simulink model "manipRotationTrajectory"  (R2019a)
settings: Solver=FixedStepAuto  StartTime=0.0  StopTime=inf  RelTol=1e-3
PreLoadFcn:
  | createWaypointData;
undefined symbols (not defined in the file): diff, gen3, maxWaypoints, ts, waypointTimes
libraries: trajExampleUtils x9, robotcorelib x4, robotmaniplib x1
settings Model: Creator=scastro  LastModifiedBy=scastro
settings DataIOCC: ReturnWorkspaceOutputs=off
settings OptimizationCC: DefaultParameterBehavior=Inlined  EnhancedBackFolding=on  PassReuseOutputArgsAs=Individual arguments  OptimizeBlockOrder=speed  DifferentSizesBufferReuse=on  OptimizationCustomize=off
settings DebuggingCC: ParameterTunabilityLossMsg=error  ArithmeticOperatorsInVariantConditions=warning
settings SFSimCC: MATLABDynamicMemAlloc=off
settings RTWCC: SystemTargetFile=ert.tlc  TemplateMakefile=ert_default_tmf  GenerateReport=on  IncludeHyperlinkInReport=on  LaunchReport=on  GenerateTraceInfo=on  GenerateTraceReport=on  GenerateTraceReportSl=on  GenerateTraceReportSf=on  GenerateTraceReportEml=on
settings CodeAppCC: ForceParamTrailComments=on  IgnoreCustomStorageClasses=off  OperatorAnnotations=on  SimulinkDataObjDesc=on  SFDataObjDesc=on  InsertBlockDesc=on
settings ERTTargetCC: TargetLangStandard=C99 (ISO)  GenerateSampleERTMain=on  SupportVariableSizeSignals=on  InlinedParameterPlacement=NonHierarchical  ERTCustomFileTemplate=example_file_process.tlc

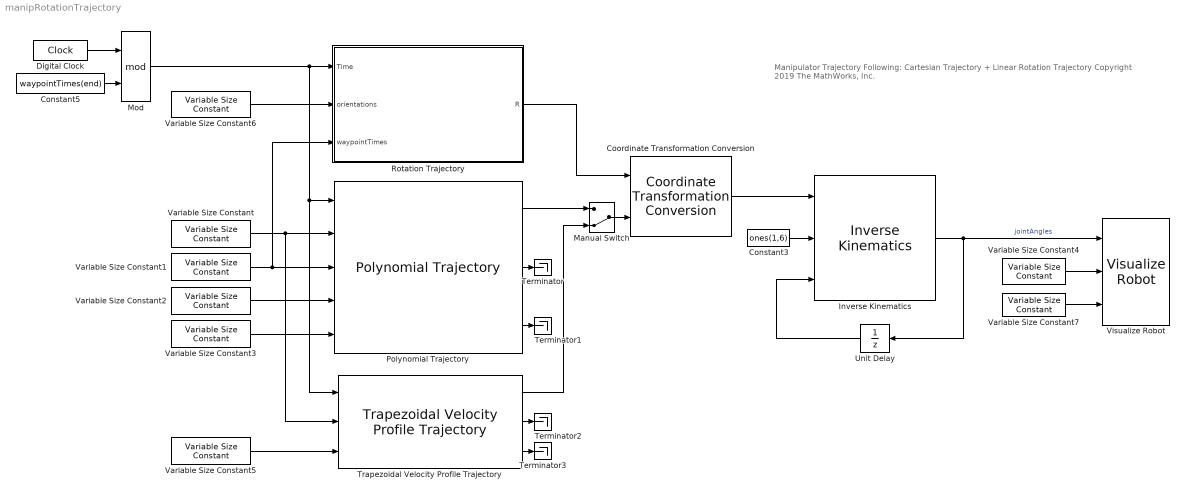
== system manipRotationTrajectory ==
  note: Manipulator Trajectory Following:
      | Cartesian Trajectory + Linear Rotation Trajectory
      |
      | Copyright 2019 The MathWorks, Inc.
  Constant3 : Constant  Value=ones(1,6)  VectorParams1D=off
  Constant5 : Constant  Value=waypointTimes(end)
  Coordinate Transformation Conversion : robotcorelib/Coordinate Transformation Conversion  InputRepresentation=Quaternion  InputEulerSequence=ZYX  ShowTrVecInputPort=on  OutputRepresentation=Homogeneous Transformation  OutputEulerSequence=ZYX  ShowTrVecOutputPort=on  SimulateUsing=Interpreted execution
      settings: SourceProductBaseCode=RO
  Digital Clock : DigitalClock  SampleTime=ts
  Inverse Kinematics : robotmaniplib/Inverse Kinematics  RigidBodyTree=gen3  EndEffector=Gripper  ShowInfo=off  SolverName=BFGS Gradient Projection  EnforceJointLimits=on  MaxIterations=1500  MaxTime=10  GradientTolerance=1e-7  SolutionTolerance=1e-6  StepTolerance=1e-14  ErrorChangeTolerance=1e-12  UseErrorDamping=on  DampingBias=0.0025  SimulateUsing=Interpreted execution
      settings: SourceProductName=Robotics System Toolbox
  Manual Switch : ManualSwitch  CurrentSetting=0
  Mod : Math  Operator=mod  SaturateOnIntegerOverflow=on
  Polynomial Trajectory : robotcorelib/Polynomial Trajectory  WaypointSource=External  Waypoints=[ 0, 2, 1, 5, 0; -1, 3, 1, 4, 4 ]  TimePoints=[ 0, 1, 2, 3, 4 ]  TimeInterval=[ 1, 4 ]  Method=Quintic Polynomial  ParameterSource=External  VelocityBoundaryCondition=zeros( 2, 5 )  AccelerationBoundaryCondition=zeros( 2, 5 )  SimulateUsing=Interpreted execution
      settings: SourceProductName=Robotics System Toolbox  SourceProductBaseCode=RO
  Rotation Trajectory : Subsystem
  Terminator{,1..3} (4 alike) : Terminator
  Trapezoidal Velocity Profile Trajectory : robotcorelib/Trapezoidal Velocity Profile Trajectory  WaypointSource=External  Waypoints=[ 0, -0.5, -1; 0, 0.5, 1 ]  NumParams=1  Parameter1=End Time  Parameter2=End Time  ParameterSource=External  PeakVelocity=[ 1; 1; 1 ]  Acceleration=[ 1; 2 ]  EndTime=[ 1; 1; 1 ]  AccelTime=[ 1; 2 ]  SimulateUsing=Interpreted execution
      settings: SourceProductName=Robotics System Toolbox  SourceProductBaseCode=RO
  Unit Delay : UnitDelay  InitialCondition=ikInitGuess'  SampleTime=-1  HasFrameUpgradeWarning=on
  Variable Size Constant : trajExampleUtils/Variable Size Constant  val=waypoints  maxSize=[3,maxWaypoints]  Ts=-1
  Variable Size Constant1 : trajExampleUtils/Variable Size Constant  val=waypointTimes  maxSize=[1,maxWaypoints]  Ts=-1
  Variable Size Constant2 : trajExampleUtils/Variable Size Constant  val=waypointVels  maxSize=[3,maxWaypoints]  Ts=-1
  Variable Size Constant3 : trajExampleUtils/Variable Size Constant  val=waypointAccels  maxSize=[3,maxWaypoints]  Ts=-1
  Variable Size Constant4 : trajExampleUtils/Variable Size Constant  val=waypoints  maxSize=[3,maxWaypoints]  Ts=-1
  Variable Size Constant5 : trajExampleUtils/Variable Size Constant  val=repmat(diff(waypointTimes),[3 1])  maxSize=[3,maxWaypoints-1]  Ts=-1
  Variable Size Constant6 : trajExampleUtils/Variable Size Constant  val=orientations  maxSize=[3,maxWaypoints]  Ts=-1
  Variable Size Constant7 : trajExampleUtils/Variable Size Constant  val=orientations  maxSize=[3,maxWaypoints]  Ts=-1
  Visualize Robot : trajExampleUtils/Visualize Robot  rbtName=gen3  eeName=Gripper  numJoints=numel(gen3.homeConfiguration)  maxPts=maxWaypoints  plotMode=Coordinate Frames
  wires:
  Digital Clock/1 -> Mod/1
  Variable Size Constant1/1 -> Rotation Trajectory/3(waypointTimes), Polynomial Trajectory/3
  Variable Size Constant2/1 -> Polynomial Trajectory/4
  Coordinate Transformation Conversion/1 -> Inverse Kinematics/1
  Constant3/1 -> Inverse Kinematics/2
  Inverse Kinematics/1 -> Visualize Robot/1, Unit Delay/1  "jointAngles"
  Mod/1 -> Rotation Trajectory/1(Time), Trapezoidal Velocity Profile Trajectory/1, Polynomial Trajectory/1
  Constant5/1 -> Mod/2
  Unit Delay/1 -> Inverse Kinematics/3
  Variable Size Constant3/1 -> Polynomial Trajectory/5
  Variable Size Constant/1 -> Trapezoidal Velocity Profile Trajectory/2, Polynomial Trajectory/2
  Polynomial Trajectory/1 -> Manual Switch/1
  Manual Switch/1 -> Coordinate Transformation Conversion/2
  Trapezoidal Velocity Profile Trajectory/1 -> Manual Switch/2
  Variable Size Constant4/1 -> Visualize Robot/2
  Rotation Trajectory/1(R) -> Coordinate Transformation Conversion/1
  Variable Size Constant6/1 -> Rotation Trajectory/2(orientations)
  Variable Size Constant5/1 -> Trapezoidal Velocity Profile Trajectory/3
  Polynomial Trajectory/2 -> Terminator/1
  Polynomial Trajectory/3 -> Terminator1/1
  Trapezoidal Velocity Profile Trajectory/2 -> Terminator2/1
  Trapezoidal Velocity Profile Trajectory/3 -> Terminator3/1
  Variable Size Constant7/1 -> Visualize Robot/3

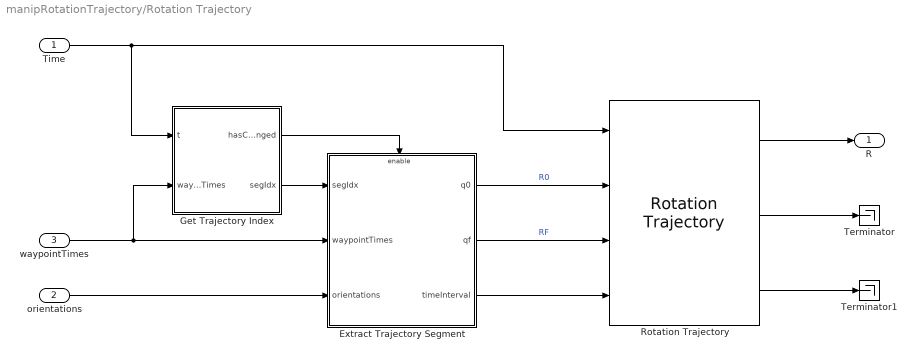
== system manipRotationTrajectory/Rotation Trajectory ==
  Time : Inport
  orientations : Inport  Port=2
  waypointTimes : Inport  Port=3
  Extract Trajectory Segment : Subsystem
  Get Trajectory Index : MATLAB Function  TreatAsAtomicUnit=on
  Rotation Trajectory : robotcorelib/Rotation Trajectory  WaypointFormat=Quaternion  WaypointSource=External  R0=[ 1, 0, 0, 0 ]'  RF=[ 0, 0, 0, 1 ]'  TimeInterval=[ 0, 4 ]  CustomTimeScaling=off  ParameterSource=Internal  TSTime=0:0.1:1  TimeScaling=[ 0:0.1:1; ones( 1, 11 ); zeros( 1, 11 ) ]  SimulateUsing=Interpreted execution
      settings: SourceProductName=Robotics System Toolbox  SourceProductBaseCode=RO
  Terminator : Terminator
  Terminator1 : Terminator
  R : Outport
  wires:
  Rotation Trajectory/1 -> R/1
  Rotation Trajectory/2 -> Terminator/1
  Rotation Trajectory/3 -> Terminator1/1
  Extract Trajectory Segment/1(q0) -> Rotation Trajectory/2  "R0"
  Extract Trajectory Segment/2(qf) -> Rotation Trajectory/3  "RF"
  Time/1 -> Get Trajectory Index/1(t), Rotation Trajectory/1
  waypointTimes/1 -> Extract Trajectory Segment/2(waypointTimes), Get Trajectory Index/2(waypointTimes)
  Get Trajectory Index/2(segIdx) -> Extract Trajectory Segment/1(segIdx)
  Get Trajectory Index/1(hasChanged) -> Extract Trajectory Segment/Enable
  Extract Trajectory Segment/3(timeInterval) -> Rotation Trajectory/4
  orientations/1 -> Extract Trajectory Segment/3(orientations)

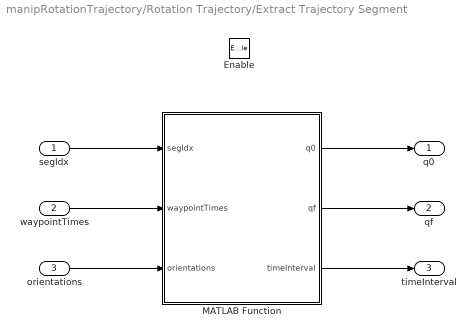
== system manipRotationTrajectory/Rotation Trajectory/Extract Trajectory Segment ==
  segIdx : Inport
  waypointTimes : Inport  Port=2
  orientations : Inport  Port=3
  Enable : EnablePort  PropagateVarSize=During execution
  MATLAB Function : MATLAB Function  TreatAsAtomicUnit=on
  q0 : Outport
  qf : Outport  Port=2
  timeInterval : Outport  Port=3
  wires:
  segIdx/1 -> MATLAB Function/1(segIdx)
  MATLAB Function/1(q0) -> q0/1
  MATLAB Function/3(timeInterval) -> timeInterval/1
  orientations/1 -> MATLAB Function/3(orientations)
  MATLAB Function/2(qf) -> qf/1
  waypointTimes/1 -> MATLAB Function/2(waypointTimes)

== matlab function manipRotationTrajectory/Rotation Trajectory/Get Trajectory Index ==
  data: hasChanged output; t input; segIdx output; waypointTimes input size=[1 maxWaypoints]
function [hasChanged,segIdx] = getTrajIdx(t,waypointTimes)

% Initialize previous index
persistent prevIdx
if isempty(prevIdx)
    prevIdx = 0;
end

% Find the trajectory segment index
segIndices = find(t>=waypointTimes);

% Limit the index value to the number of times minus one
% (This addresses the final time case)
segIdx = min(segIndices(end),numel(waypointTimes)-1);

% Determine whether the index has changed from the previous time step
if prevIdx == segIdx
    hasChanged = false;
else
    hasChanged = true;
    prevIdx = segIdx;
end

end

== matlab function manipRotationTrajectory/Rotation Trajectory/Extract Trajectory Segment/MATLAB Function ==
  data: segIdx input; waypointTimes input size=[1 maxWaypoints]; q0 output size=[1 4]; orientations input size=[3 maxWaypoints]; qf output size=[1 4]; timeInterval output size=[1 2]
function [q0, qf, timeInterval] = createRotationTrajSegment(segIdx,waypointTimes,orientations)

% Extract the time interval, initial, and final quaternions for the segment
timeInterval = waypointTimes(segIdx:segIdx+1);
q0 = eul2quat(orientations(:,segIdx)');
qf = eul2quat(orientations(:,segIdx+1)');

end
